simulink subsystem "VehicleElectroThermal"  (R2023a)
settings: Solver=VariableStepAuto  StartTime=0.0  StopTime=10.0  RelTol=1e-3
undefined symbols (not defined in the file): battery, cabin_T_init, coolant_pipe_D, coolant_valve_D_ratio_max, coolant_valve_D_ratio_min, coolant_valve_displacement, vehicleThermal
libraries: fl_lib x199, nesl_utility x54, SimscapeFluids_lib x15, ee_lib x9, sdl_lib x8, slpidlib x3, simulink x2, EmotorLib x2, BatteryCurrentManagement x1
(part 1 of 6)
settings Model: Creator=jjha  LastModifiedBy=jjha
settings OptimizationCC: ReuseModelBlockBuffer=off

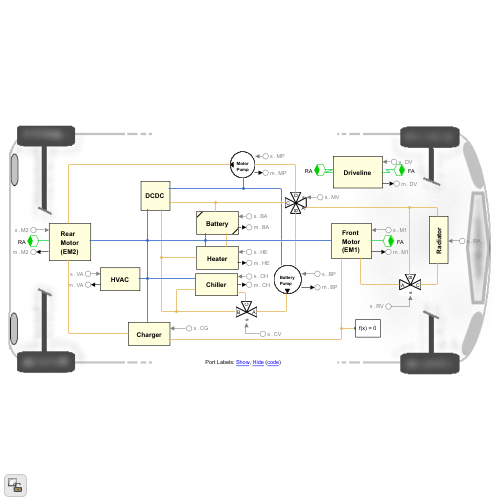
[thumbnail: Simulink's stored preview of the top-level diagram]
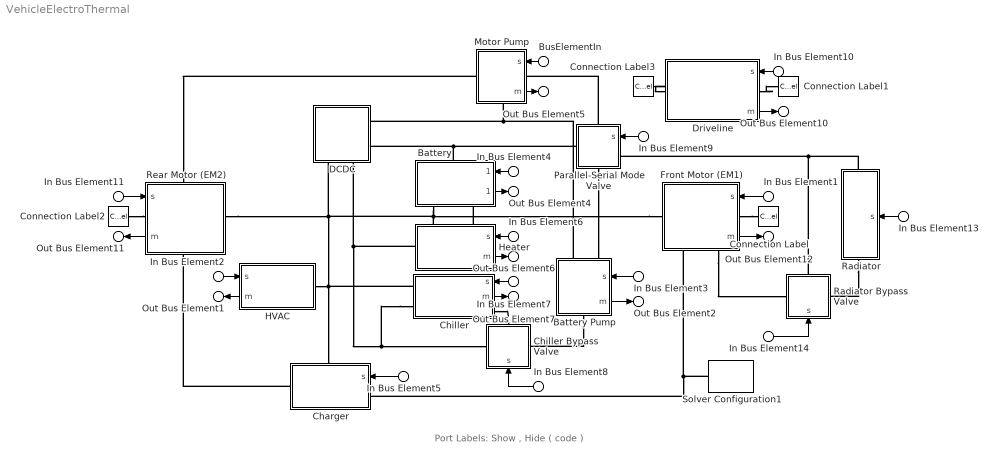
== system VehicleElectroThermal ==
  note: Port Labels: Show , Hide ( code )
  In Bus Element2 : Inport  PortName=s  Element=VA
  In Bus Element3 : Inport  PortName=s  Element=BP
  In Bus Element4 : Inport  PortName=s  Element=BA
  In Bus Element6 : Inport  PortName=s  Element=HE
  In Bus Element7 : Inport  PortName=s  Element=CH
  In Bus Element8 : Inport  PortName=s  Element=CV
  In Bus Element9 : Inport  PortName=s  Element=MV
  In Bus Element10 : Inport  PortName=s  Element=DV
  In Bus Element11 : Inport  PortName=s  Element=M2
  In Bus Element13 : Inport  PortName=s  Element=RA
  In Bus Element14 : Inport  PortName=s  Element=RV
  BusElementIn : Inport  PortName=s  Element=MP
  In Bus Element5 : Inport  PortName=s  Element=CG
  In Bus Element1 : Inport  PortName=s  Element=M1
  Battery : Subsystem  ReferencedSubsystem=BatteryPlantModelLumped_th
      settings: PortSchema="{\"entries\":[{\"content\":{\"sides\":[{\"content\":{\"connectorIds\":[\"In1\",\"Out1\"]},\"type\":\"ConnectorPlacement.EquallySpacedRectSide\",\"uuid\":\"8937d0fc-2bf4-4b6f-a857-82b384a76c94\"},{\"content\":{\"side\":\"RIGHT\"},\"type\":\"ConnectorPlacement.EquallySpacedRectSide\",\"uuid\":\"1ccbeec6-a013-4076-9f98-cb308866a19c\"},{\"content\":{\"connectorIds\":[\"LConn1\"],\"side\":\"TOP\"},\"type\":\"ConnectorPlacement.EquallySpacedRectSide\",\"uuid\":\"77a454e3-c37c-480e-9dd0-9550186f5eb3\"},{\"content\":{\"connectorIds\":[\"RConn1\",\"RConn2\"],\"side\":\"BOTTOM\"},\"type\":\"ConnectorPlacement.EquallySpacedRectSide\",\"uuid\":\"f9a87c6a-7374-41c2-a5df-89d60c915a70\"}]},\"type\":\"ConnectorPlacement.EquallySpacedConnector\",\"uuid\":\"fe008494-fd6d-45a8-bf6b-36872afbad95\"}],\"packageUris\":[\"http://schema.mathworks.com/mf0/Connector/R2020b\"],\"version\":\"1.0\"}"
  Battery Pump : Subsystem  Tag=PublishSubsystem
      settings: PortSchema="{\"entries\":[{\"content\":{\"sides\":[{\"content\":{\"connectorIds\":[\"In1\",\"Out1\"]},\"type\":\"ConnectorPlacement.EquallySpacedRectSide\",\"uuid\":\"f321ff85-78a4-45a4-ab97-f20c5abfaf5e\"},{\"content\":{\"connectorIds\":[],\"side\":\"RIGHT\"},\"type\":\"ConnectorPlacement.EquallySpacedRectSide\",\"uuid\":\"2baf3540-3ef2-4140-8c68-0a1895e3ee25\"},{\"content\":{\"connectorIds\":[\"LConn1\",\"LConn2\"],\"side\":\"TOP\"},\"type\":\"ConnectorPlacement.EquallySpacedRectSide\",\"uuid\":\"1e5b09ba-71c5-41d6-b265-2fb2d783e941\"},{\"content\":{\"connectorIds\":[\"RConn1\"],\"side\":\"BOTTOM\"},\"type\":\"ConnectorPlacement.EquallySpacedRectSide\",\"uuid\":\"998b9f49-32fc-4a08-8ed4-02bb722e6368\"}]},\"type\":\"ConnectorPlacement.EquallySpacedConnector\",\"uuid\":\"4c01441a-ee4a-4858-900a-4caacc6910c3\"}],\"packageUris\":[\"http://schema.mathworks.com/mf0/Connector/R2020b\"],\"version\":\"1.0\"}"
      mask Display:
      | plot(150*cos(linspace(0, 2*pi, 500)), 150*sin(linspace(0, 2*pi, 500)))
      | patch([0 24 -24 0],-1*([100 55 55 100]-1+50),  [0 0 0])
      | %disp(get_param(gcb, 'Name'))
      | disp(['{\bf\fontsize{8}' get_param(gcb, 'Name') '}'], 'texmode','on');
  Charger : Subsystem
      settings: PortSchema="{\"entries\":[{\"content\":{\"sides\":[{\"content\":{\"connectorIds\":[\"In1\",\"LConn1\"]},\"type\":\"ConnectorPlacement.EquallySpacedRectSide\",\"uuid\":\"cb45011f-5d5d-4b7e-92e7-7d115d1e4fd6\"},{\"content\":{\"connectorIds\":[\"RConn1\"],\"side\":\"RIGHT\"},\"type\":\"ConnectorPlacement.EquallySpacedRectSide\",\"uuid\":\"cd67087d-6bbf-411e-9f50-cc3c1f5fce85\"},{\"content\":{\"connectorIds\":[\"LConn2\"],\"side\":\"TOP\"},\"type\":\"ConnectorPlacement.EquallySpacedRectSide\",\"uuid\":\"32ff64c9-862a-431f-9f24-2baf455cdab5\"}]},\"type\":\"ConnectorPlacement.EquallySpacedConnector\",\"uuid\":\"13ffd7d0-36a1-4766-a9dc-2d010b2a8713\"}],\"packageUris\":[\"http://schema.mathworks.com/mf0/Connector/R2020b\"],\"version\":\"1.0\"}"
      mask Display:
      | %disp(get_param(gcb, 'Name'))
      | disp(['{\bf\fontsize{12}' get_param(gcb, 'Name') '}'], 'texmode','on');
  Chiller : Subsystem
      settings: PortSchema="{\"entries\":[{\"content\":{\"sides\":[{\"content\":{\"connectorIds\":[\"LConn1\",\"LConn2\"]},\"type\":\"ConnectorPlacement.EquallySpacedRectSide\",\"uuid\":\"5c01cf01-1aa7-4ead-a658-6b31c847d37c\"},{\"content\":{\"connectorIds\":[\"In1\",\"Out1\",\"RConn1\"],\"side\":\"RIGHT\"},\"type\":\"ConnectorPlacement.EquallySpacedRectSide\",\"uuid\":\"fa598d46-0793-4efa-a9e2-c958f5dfdee6\"},{\"content\":{\"connectorIds\":[],\"side\":\"TOP\"},\"type\":\"ConnectorPlacement.EquallySpacedRectSide\",\"uuid\":\"e82d971a-2580-41ee-87fa-0ab5603b5665\"},{\"content\":{\"connectorIds\":[],\"side\":\"BOTTOM\"},\"type\":\"ConnectorPlacement.EquallySpacedRectSide\",\"uuid\":\"431a910f-738f-40ab-a4d4-f974d0793b92\"}]},\"type\":\"ConnectorPlacement.EquallySpacedConnector\",\"uuid\":\"9f63eeb1-1768-47e0-a5e5-2e43c100d3fd\"}],\"packageUris\":[\"http://schema.mathworks.com/mf0/Connector/R2020b\"],\"version\":\"1.0\"}"
      mask Display:
      | %disp(get_param(gcb, 'Name'))
      | disp(['{\bf\fontsize{12}' get_param(gcb, 'Name') '}'], 'texmode','on');
  Chiller Bypass Valve : Subsystem  Tag=PublishSubsystem
      settings: PortSchema="{\"entries\":[{\"content\":{\"sides\":[{\"content\":{\"connectorIds\":[\"LConn1\"]},\"type\":\"ConnectorPlacement.EquallySpacedRectSide\",\"uuid\":\"3cf8f321-e6af-4e16-922c-cceb23b0b295\"},{\"content\":{\"connectorIds\":[\"In1\"],\"side\":\"RIGHT\"},\"type\":\"ConnectorPlacement.EquallySpacedRectSide\",\"uuid\":\"d134eacd-e7eb-4b63-940a-90eaf4978625\"},{\"content\":{\"connectorIds\":[\"LConn2\"],\"side\":\"TOP\"},\"type\":\"ConnectorPlacement.EquallySpacedRectSide\",\"uuid\":\"57a3d5f7-3b46-4166-b258-196ae00f6810\"},{\"content\":{\"connectorIds\":[\"RConn1\"],\"side\":\"BOTTOM\"},\"type\":\"ConnectorPlacement.EquallySpacedRectSide\",\"uuid\":\"637149da-33c2-49a6-af44-c757a7002402\"}]},\"type\":\"ConnectorPlacement.EquallySpacedConnector\",\"uuid\":\"8ee22012-655b-4352-9f09-996f74687633\"}],\"packageUris\":[\"http://schema.mathworks.com/mf0/Connector/R2020b\"],\"version\":\"1.0\"}"
      mask Display:
      | color('white')
      | plot(100, 100)
      | plot(-100, -100)
      | color('black')
      | 
      | plot([0 -100 -100 0], [0 50 -50 0])
      | plot([0 50 -50 0], [0 100 100 0])
      | plot([0 50 -50 0], [0 -100 -100 0])
  Connection Label : ConnectionLabel  Label=FA
  Connection Label1 : ConnectionLabel  Label=FA
  Connection Label2 : ConnectionLabel  Label=RA
  Connection Label3 : ConnectionLabel  Label=RA
  DCDC : Subsystem
      settings: PortSchema="{\"entries\":[{\"content\":{\"sides\":[{\"content\":{},\"type\":\"ConnectorPlacement.EquallySpacedRectSide\",\"uuid\":\"88f70306-1074-4a2f-bf6e-5266a6fad5cc\"},{\"content\":{\"connectorIds\":[\"RConn1\",\"RConn2\"],\"side\":\"RIGHT\"},\"type\":\"ConnectorPlacement.EquallySpacedRectSide\",\"uuid\":\"c9954f31-88d1-45ba-bccc-746174ca97ad\"},{\"content\":{\"side\":\"TOP\"},\"type\":\"ConnectorPlacement.EquallySpacedRectSide\",\"uuid\":\"3d242faa-6d27-4f03-9691-d9501eee9202\"},{\"content\":{\"connectorIds\":[\"RConn3\",\"RConn4\"],\"side\":\"BOTTOM\"},\"type\":\"ConnectorPlacement.EquallySpacedRectSide\",\"uuid\":\"dbc5cd88-c0c4-43cc-b68d-d7b9b93e8ccf\"}]},\"type\":\"ConnectorPlacement.EquallySpacedConnector\",\"uuid\":\"8b73b678-f81c-41f4-a7f6-152147edfd1f\"}],\"packageUris\":[\"http://schema.mathworks.com/mf0/Connector/R2020b\"],\"version\":\"1.0\"}"
      mask Display:
      | %disp(get_param(gcb, 'Name'))
      | disp(['{\bf\fontsize{12}' get_param(gcb, 'Name') '}'], 'texmode','on');
  Driveline : Subsystem
      settings: PortSchema="{\"entries\":[{\"content\":{\"sides\":[{\"content\":{\"connectorIds\":[\"In1\",\"LConn1\",\"Out1\"]},\"type\":\"ConnectorPlacement.EquallySpacedRectSide\",\"uuid\":\"f321ff85-78a4-45a4-ab97-f20c5abfaf5e\"},{\"content\":{\"connectorIds\":[\"RConn1\"],\"side\":\"RIGHT\"},\"type\":\"ConnectorPlacement.EquallySpacedRectSide\",\"uuid\":\"2baf3540-3ef2-4140-8c68-0a1895e3ee25\"},{\"content\":{\"connectorIds\":[],\"side\":\"TOP\"},\"type\":\"ConnectorPlacement.EquallySpacedRectSide\",\"uuid\":\"1e5b09ba-71c5-41d6-b265-2fb2d783e941\"}]},\"type\":\"ConnectorPlacement.EquallySpacedConnector\",\"uuid\":\"4c01441a-ee4a-4858-900a-4caacc6910c3\"}],\"packageUris\":[\"http://schema.mathworks.com/mf0/Connector/R2020b\"],\"version\":\"1.0\"}"
      mask Display:
      | %disp(get_param(gcb, 'Name'))
      | disp(['{\bf\fontsize{12}' get_param(gcb, 'Name') '}'], 'texmode','on');
  Front Motor (EM1) : Subsystem
      settings: PortSchema="{\"entries\":[{\"content\":{\"sides\":[{\"content\":{\"connectorIds\":[\"In1\",\"LConn1\",\"Out1\"]},\"type\":\"ConnectorPlacement.EquallySpacedRectSide\",\"uuid\":\"7243fc6e-711d-4968-986e-a6ac860e50c1\"},{\"content\":{\"connectorIds\":[\"RConn1\"],\"side\":\"RIGHT\"},\"type\":\"ConnectorPlacement.EquallySpacedRectSide\",\"uuid\":\"18479f7a-8f27-458a-ae71-b38762574ae4\"},{\"content\":{\"connectorIds\":[],\"side\":\"TOP\"},\"type\":\"ConnectorPlacement.EquallySpacedRectSide\",\"uuid\":\"aa936f76-6865-41c5-8414-293bd7d656ce\"},{\"content\":{\"connectorIds\":[\"RConn2\",\"RConn3\"],\"side\":\"BOTTOM\"},\"type\":\"ConnectorPlacement.EquallySpacedRectSide\",\"uuid\":\"336e35a4-9a9a-4631-a8f5-a4d8b8cf9e70\"}]},\"type\":\"ConnectorPlacement.EquallySpacedConnector\",\"uuid\":\"faab3502-7b69-46ce-a6d2-3155f4c3b486\"}],\"packageUris\":[\"http://schema.mathworks.com/mf0/Connector/R2020b\"],\"version\":\"1.0\"}"
      mask Display:
      | %disp(get_param(gcb, 'Name'))
      | disp(['{\bf\fontsize{12}' get_param(gcb, 'Name') '}'], 'texmode','on');
  HVAC : Subsystem
      settings: PortSchema="{\"entries\":[{\"content\":{\"sides\":[{\"content\":{\"connectorIds\":[\"LConn1\"]},\"type\":\"ConnectorPlacement.EquallySpacedRectSide\",\"uuid\":\"f3199610-b7b9-4772-9d43-f46decbe6ee9\"},{\"content\":{\"connectorIds\":[\"In1\",\"Out1\"],\"side\":\"RIGHT\"},\"type\":\"ConnectorPlacement.EquallySpacedRectSide\",\"uuid\":\"92399d3a-435b-4545-8fb9-2408b0c62154\"},{\"content\":{\"connectorIds\":[],\"side\":\"TOP\"},\"type\":\"ConnectorPlacement.EquallySpacedRectSide\",\"uuid\":\"9d5257be-bcde-46da-a005-cbe35149e50d\"},{\"content\":{\"connectorIds\":[],\"side\":\"BOTTOM\"},\"type\":\"ConnectorPlacement.EquallySpacedRectSide\",\"uuid\":\"da7f19de-1e57-4fc2-b5c3-4c1d680ac086\"}]},\"type\":\"ConnectorPlacement.EquallySpacedConnector\",\"uuid\":\"aa27bbb1-a774-4836-83ea-faf9e12779cd\"}],\"packageUris\":[\"http://schema.mathworks.com/mf0/Connector/R2020b\"],\"version\":\"1.0\"}"
      mask Display:
      | %disp(get_param(gcb, 'Name'))
      | disp(['{\bf\fontsize{12}' get_param(gcb, 'Name') '}'], 'texmode','on');
  Heater : Subsystem
      settings: PortSchema="{\"entries\":[{\"content\":{\"sides\":[{\"content\":{\"connectorIds\":[]},\"type\":\"ConnectorPlacement.EquallySpacedRectSide\",\"uuid\":\"f321ff85-78a4-45a4-ab97-f20c5abfaf5e\"},{\"content\":{\"connectorIds\":[\"RConn1\",\"RConn2\"],\"side\":\"RIGHT\"},\"type\":\"ConnectorPlacement.EquallySpacedRectSide\",\"uuid\":\"2baf3540-3ef2-4140-8c68-0a1895e3ee25\"},{\"content\":{\"connectorIds\":[\"Out1\",\"In1\"],\"side\":\"TOP\"},\"type\":\"ConnectorPlacement.EquallySpacedRectSide\",\"uuid\":\"1e5b09ba-71c5-41d6-b265-2fb2d783e941\"},{\"content\":{\"connectorIds\":[\"RConn3\"],\"side\":\"BOTTOM\"},\"type\":\"ConnectorPlacement.EquallySpacedRectSide\",\"uuid\":\"2993c442-350f-4391-ac34-e98798b669d5\"}]},\"type\":\"ConnectorPlacement.EquallySpacedConnector\",\"uuid\":\"4c01441a-ee4a-4858-900a-4caacc6910c3\"}],\"packageUris\":[\"http://schema.mathworks.com/mf0/Connector/R2020b\"],\"version\":\"1.0\"}"
      mask Display:
      | %disp(get_param(gcb, 'Name'))
      | disp(['{\bf\fontsize{12}' get_param(gcb, 'Name') '}'], 'texmode','on');
  Motor Pump : Subsystem  Tag=PublishSubsystem
      settings: PortSchema="{\"entries\":[{\"content\":{\"sides\":[{\"content\":{\"connectorIds\":[\"In1\",\"LConn1\",\"Out1\"]},\"type\":\"ConnectorPlacement.EquallySpacedRectSide\",\"uuid\":\"dafa5c41-979f-4f2b-beb0-03378b6030c3\"},{\"content\":{\"connectorIds\":[\"RConn1\"],\"side\":\"RIGHT\"},\"type\":\"ConnectorPlacement.EquallySpacedRectSide\",\"uuid\":\"2ea2b4cc-bcb0-4b93-915b-9928efecd2a3\"},{\"content\":{\"connectorIds\":[],\"side\":\"TOP\"},\"type\":\"ConnectorPlacement.EquallySpacedRectSide\",\"uuid\":\"e510a9c0-a763-4750-a71a-9698d7ffd631\"},{\"content\":{\"connectorIds\":[\"RConn2\"],\"side\":\"BOTTOM\"},\"type\":\"ConnectorPlacement.EquallySpacedRectSide\",\"uuid\":\"6a9cd967-74c4-4a03-9c08-7c7b4b09ecc0\"}]},\"type\":\"ConnectorPlacement.EquallySpacedConnector\",\"uuid\":\"4a878def-b7f5-448f-823c-c871001bb196\"}],\"packageUris\":[\"http://schema.mathworks.com/mf0/Connector/R2020b\"],\"version\":\"1.0\"}"
      mask Display:
      | plot(150*cos(linspace(0, 2*pi, 500)), 150*sin(linspace(0, 2*pi, 500)))
      | patch([-100 -55 -55 -100]-50, [0 24 -24 0], [0 0 0])
      | %disp(get_param(gcb, 'Name'))
      | disp(['{\bf\fontsize{8}' get_param(gcb, 'Name') '}'], 'texmode','on');
  Parallel-Serial Mode Valve : Subsystem  Tag=PublishSubsystem
      settings: PortSchema="{\"entries\":[{\"content\":{\"sides\":[{\"content\":{\"connectorIds\":[\"LConn1\"]},\"type\":\"ConnectorPlacement.EquallySpacedRectSide\",\"uuid\":\"37aeff26-8a07-411b-9eeb-30a57d0de01e\"},{\"content\":{\"connectorIds\":[\"RConn1\"],\"side\":\"RIGHT\"},\"type\":\"ConnectorPlacement.EquallySpacedRectSide\",\"uuid\":\"5bec464c-49bf-4ce7-bef9-f1dcc380cec5\"},{\"content\":{\"connectorIds\":[\"LConn2\",\"In1\"],\"side\":\"TOP\"},\"type\":\"ConnectorPlacement.EquallySpacedRectSide\",\"uuid\":\"af2a9b5d-b1fd-40d4-a7a1-24f37b8a323f\"},{\"content\":{\"connectorIds\":[\"RConn2\"],\"side\":\"BOTTOM\"},\"type\":\"ConnectorPlacement.EquallySpacedRectSide\",\"uuid\":\"7361a3ef-1473-4ec0-bd8f-80e79015a6c8\"}]},\"type\":\"ConnectorPlacement.EquallySpacedConnector\",\"uuid\":\"019cf393-57f8-4763-b38e-2892ad46a0e9\"}],\"packageUris\":[\"http://schema.mathworks.com/mf0/Connector/R2020b\"],\"version\":\"1.0\"}"
      mask Display:
      | color('white')
      | plot(100, 100)
      | plot(-100, -100)
      | color('black')
      | 
      | plot([0 -100 -100 0], [0 50 -50 0])
      | plot([0 100 100 0], [0 50 -50 0])
      | plot([0 50 -50 0], [0 100 100 0])
      | plot([0 50 -50 0], [0 -100 -100 0])
  Radiator : Subsystem  Tag=PublishSubsystem
      settings: PortSchema="{\"entries\":[{\"content\":{\"sides\":[{\"content\":{\"connectorIds\":[\"LConn1\"]},\"type\":\"ConnectorPlacement.EquallySpacedRectSide\",\"uuid\":\"f321ff85-78a4-45a4-ab97-f20c5abfaf5e\"},{\"content\":{\"connectorIds\":[\"RConn1\"],\"side\":\"RIGHT\"},\"type\":\"ConnectorPlacement.EquallySpacedRectSide\",\"uuid\":\"2baf3540-3ef2-4140-8c68-0a1895e3ee25\"},{\"content\":{\"connectorIds\":[],\"side\":\"TOP\"},\"type\":\"ConnectorPlacement.EquallySpacedRectSide\",\"uuid\":\"1e5b09ba-71c5-41d6-b265-2fb2d783e941\"},{\"content\":{\"connectorIds\":[\"In1\"],\"side\":\"BOTTOM\"},\"type\":\"ConnectorPlacement.EquallySpacedRectSide\",\"uuid\":\"c5239a7c-78e5-4ad8-9ce6-8204a250a1f6\"}]},\"type\":\"ConnectorPlacement.EquallySpacedConnector\",\"uuid\":\"4c01441a-ee4a-4858-900a-4caacc6910c3\"}],\"packageUris\":[\"http://schema.mathworks.com/mf0/Connector/R2020b\"],\"version\":\"1.0\"}"
      mask Display:
      | %disp(get_param(gcb, 'Name'))
      | disp(['{\bf\fontsize{12}' get_param(gcb, 'Name') '}'], 'texmode','on');
  Radiator Bypass Valve : Subsystem  Tag=PublishSubsystem
      settings: PortSchema="{\"entries\":[{\"content\":{\"sides\":[{\"content\":{\"connectorIds\":[\"LConn1\"]},\"type\":\"ConnectorPlacement.EquallySpacedRectSide\",\"uuid\":\"3cf8f321-e6af-4e16-922c-cceb23b0b295\"},{\"content\":{\"connectorIds\":[\"In1\"],\"side\":\"RIGHT\"},\"type\":\"ConnectorPlacement.EquallySpacedRectSide\",\"uuid\":\"d134eacd-e7eb-4b63-940a-90eaf4978625\"},{\"content\":{\"connectorIds\":[\"LConn2\"],\"side\":\"TOP\"},\"type\":\"ConnectorPlacement.EquallySpacedRectSide\",\"uuid\":\"57a3d5f7-3b46-4166-b258-196ae00f6810\"},{\"content\":{\"connectorIds\":[\"RConn1\"],\"side\":\"BOTTOM\"},\"type\":\"ConnectorPlacement.EquallySpacedRectSide\",\"uuid\":\"f8aa24a3-5169-478a-b161-4d226dc0f508\"}]},\"type\":\"ConnectorPlacement.EquallySpacedConnector\",\"uuid\":\"8ee22012-655b-4352-9f09-996f74687633\"}],\"packageUris\":[\"http://schema.mathworks.com/mf0/Connector/R2020b\"],\"version\":\"1.0\"}"
      mask Display:
      | color('white')
      | plot(100, 100)
      | plot(-100, -100)
      | color('black')
      | 
      | plot([0 -100 -100 0], [0 50 -50 0])
      | plot([0 50 -50 0], [0 100 100 0])
      | plot([0 50 -50 0], [0 -100 -100 0])
  Rear Motor (EM2) : Subsystem
      settings: PortSchema="{\"entries\":[{\"content\":{\"sides\":[{\"content\":{\"connectorIds\":[\"LConn1\"]},\"type\":\"ConnectorPlacement.EquallySpacedRectSide\",\"uuid\":\"50b93907-dab5-4c80-8f3d-b9696f7ba561\"},{\"content\":{\"connectorIds\":[\"In1\",\"RConn1\",\"Out1\"],\"side\":\"RIGHT\"},\"type\":\"ConnectorPlacement.EquallySpacedRectSide\",\"uuid\":\"ca5b0fd2-80b7-4a93-a409-39e052d42ed0\"},{\"content\":{\"connectorIds\":[\"LConn2\"],\"side\":\"TOP\"},\"type\":\"ConnectorPlacement.EquallySpacedRectSide\",\"uuid\":\"a20c906c-aee3-4b84-9c3f-344dbfe549ed\"},{\"content\":{\"connectorIds\":[\"RConn2\"],\"side\":\"BOTTOM\"},\"type\":\"ConnectorPlacement.EquallySpacedRectSide\",\"uuid\":\"c8c8c4b4-9dd9-46bd-a7c0-676d6e20cefe\"}]},\"type\":\"ConnectorPlacement.EquallySpacedConnector\",\"uuid\":\"5e07fad4-8c29-4119-b1ea-c96ebc59433e\"}],\"packageUris\":[\"http://schema.mathworks.com/mf0/Connector/R2020b\"],\"version\":\"1.0\"}"
      mask Display:
      | %disp(get_param(gcb, 'Name'))
      | disp(['{\bf\fontsize{12}' get_param(gcb, 'Name') '}'], 'texmode','on');
  Solver Configuration1 : nesl_utility/Solver Configuration  PhysicalDomain=network_engine_domain  SubClassName=solver  LeftPortType=input  RightPortType=generic  Tones=[]  Harmonics=[]  SimulateNoise=off  Profile=off  UseLocalSampling=off  EnableSwitchedLinearOptims=on  FrequencyDomain=off  UseCCode=off  RelTol=0.001  AbsTol=0.001  MinStep=1e-09  ToWorkspace=off  RevertToSquareIcSolve=off  NumHomotopyIterations=100  PhasorMode=off  PhasorModeNumHarmonics=1  ConsistencySolver=NEWTON_XTOL_AFTER_FTOL  IndexReductionMethod=DerivativeReplacement  DoDC=off  ResidualTolerance=1e-09  ConsistencyTolSource=GLOBAL  ConsistencyAbsTol=0.001  ConsistencyRelTol=0.001  ConsistencyTolFactor=0.001  UseLocalSolver=off  LocalSolverChoice=NE_BACKWARD_EULER_ADVANCER  ResolveIndetEquations=on  FunctionEvalNumThread=1  LocalSolverSampleTime=0.001  DoFixedCost=off  MaxNonlinIter=3  MaxModeIter=2  ComputeImpulses=off  ImpulseIterations=2  LinearAlgebra=auto  LinearAlgebraNumThread=0  EquationFormulation=NE_TIME_EF  DelaysMemoryBudget=1024  AutomaticFiltering=on  FilteringTimeConstant=0.001  PartitionStorageMethod=AS_NEEDED  PartitionMemoryBudget=1024  PartitionMethod=ROBUST
  Out Bus Element1 : Outport  PortName=m  Element=VA
  Out Bus Element2 : Outport  PortName=m  Element=BP
  Out Bus Element4 : Outport  PortName=m  Element=BA
  Out Bus Element6 : Outport  PortName=m  Element=HE
  Out Bus Element7 : Outport  PortName=m  Element=CH
  Out Bus Element10 : Outport  PortName=m  Element=DV
  Out Bus Element11 : Outport  PortName=m  Element=M2
  Out Bus Element12 : Outport  PortName=m  Element=M1
  Out Bus Element5 : Outport  PortName=m  Element=MP
  wires:
  In Bus Element2/1 -> HVAC/1(s)
  In Bus Element6/1 -> Heater/1(s)
  In Bus Element4/1 -> Battery/1
  Chiller/1(m) -> Out Bus Element7/1
  In Bus Element7/1 -> Chiller/1(s)
  Battery Pump/1("  m ") -> Out Bus Element2/1
  BusElementIn/1 -> Motor Pump/1(s)
  In Bus Element3/1 -> Battery Pump/1(s)
  Battery/1 -> Out Bus Element4/1
  HVAC/1(m) -> Out Bus Element1/1
  In Bus Element8/1 -> Chiller Bypass Valve/1(s)
  In Bus Element9/1 -> Parallel-Serial Mode Valve/1(s)
  Driveline/1(m) -> Out Bus Element10/1
  In Bus Element10/1 -> Driveline/1(s)
  In Bus Element11/1 -> Rear Motor (EM2)/1(s)
  Rear Motor (EM2)/1(m) -> Out Bus Element11/1
  Front Motor (EM1)/1(m) -> Out Bus Element12/1
  In Bus Element13/1 -> Radiator/1(s)
  In Bus Element14/1 -> Radiator Bypass Valve/1(s)
  In Bus Element5/1 -> Charger/1(s)
  Heater/1(m) -> Out Bus Element6/1
  Motor Pump/1("  m ") -> Out Bus Element5/1
  In Bus Element1/1 -> Front Motor (EM1)/1(s)
  connections:
  Parallel-Serial Mode Valve/LConn2 -- Radiator/RConn1 -- Radiator Bypass Valve/LConn1
  Charger/LConn1 -- Front Motor (EM1)/RConn3 -- Solver Configuration1/RConn1
  Chiller/LConn2 -- Heater/RConn3 -- DCDC/RConn4 -- Chiller Bypass Valve/RConn1
  Parallel-Serial Mode Valve/RConn2 -- DCDC/RConn2 -- Battery/LConn1
  Front Motor (EM1)/RConn1 -- Charger/LConn2 -- HVAC/LConn1 -- Chiller/LConn1 -- Rear Motor (EM2)/LConn1 -- DCDC/RConn3 -- Battery/RConn2 -- Heater/RConn2
  Battery Pump/LConn2 -- Motor Pump/RConn2 -- DCDC/RConn1
  Battery Pump/RConn1 -- Chiller Bypass Valve/LConn2
  Parallel-Serial Mode Valve/RConn1 -- Motor Pump/LConn1
  Motor Pump/RConn1 -- Rear Motor (EM2)/LConn2
  Parallel-Serial Mode Valve/LConn1 -- Battery Pump/LConn1
  Charger/RConn1 -- Rear Motor (EM2)/RConn2
  Connection Label2/LConn1 -- Rear Motor (EM2)/RConn1
  Front Motor (EM1)/LConn1 -- Connection Label/LConn1
  Chiller/RConn1 -- Chiller Bypass Valve/LConn1
  Radiator/LConn1 -- Radiator Bypass Valve/RConn1
  Front Motor (EM1)/RConn2 -- Radiator Bypass Valve/LConn2
  Driveline/LConn1 -- Connection Label1/LConn1
  Connection Label3/LConn1 -- Driveline/RConn1
  Heater/RConn1 -- Battery/RConn1

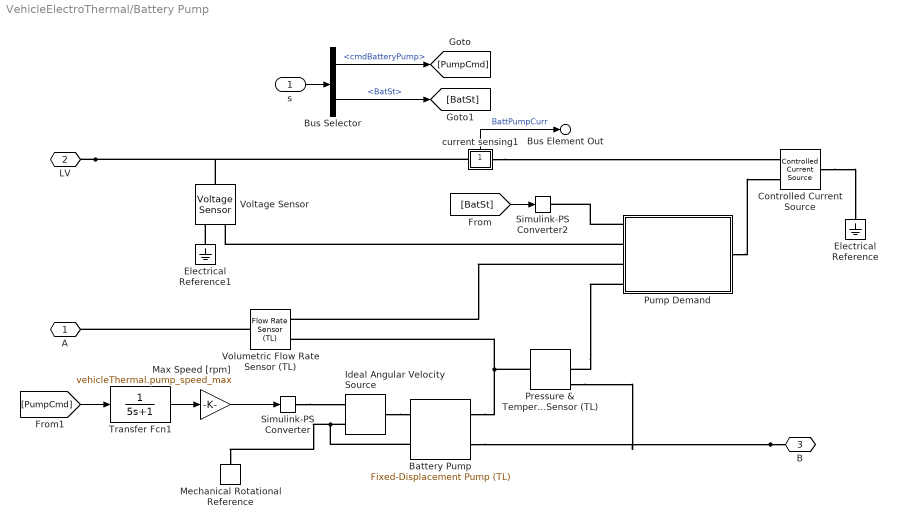
== system VehicleElectroThermal/Battery Pump ==
  s : Inport
  Battery Pump : SimscapeFluids_lib/Thermal Liquid/Pumps & Motors/Fixed-Displacement Pump (TL)  loss_spec=1  displacement=vehicleThermal.pump_displacement l/rev  omega_nominal=0.5 * vehicleThermal.pump_speed_max rpm  p_nominal=0.1 MPa  mu_nominal=0.9 cP  vol_eff_nominal=0.92  mech_eff_nominal=1/(1 + (0.6)/(vehicleThermal.pump_displacement)*0.006283185307179586 + (0.05)/(vehicleThermal.pump_displacement)/(0.1)*0.006283185307179586)  no_load_torque=0.05 N*m  p_diff_eff_TLU=[.1, 1, 2] MPa  omega_eff_TLU=[25, 50, 100, 200, 300, 400] rad/s  vol_eff_TLU=[.816, .908, .954, .977, .981, .984; .325, .663, .831, .916, .925, .946; .137, .568, .78, .892, .893, .91]  mech_eff_TLU=[.996, .996, .996, .996, .996, .996; .988, .989, .989, .989, .989, .99; .981, .981, .982, .982, .983, .984]  p_diff_loss_TLU=[.1, 1, 2] MPa  omega_loss_TLU=[25, 50, 100, 200, 300, 400] rad/s  vol_loss_TLU=[.023, .023, .023, .023, .0285, .032; .0844, .0842, .0845, .084, .1125, .108; .1079, .108, .11, .108, .1605, .18] * 1e-3 m^3/s  mech_loss_TLU=[.002, .002, .002, .002, .002, .002; .0607, .0556, .0556, .0556, .0556, .0505; .1937, .1937, .1833, .1833, .1729, .1626] N*m  vol_eff_min=1e-3  vol_eff_max=1  mech_eff_min=1e-3  mech_eff_max=1  pressure_threshold=1e-3 MPa  omega_threshold=10 rad/s  area=pi * vehicleThermal.coolant_pipe_D^2 / 4 m^2  quadrant_check=0  pump_mode_check=simscape.enum.assert.action.none
  Bus Selector : BusSelector  OutputSignals=cmdBatteryPump,BatSt
  Controlled Current Source : fl_lib/Electrical/Electrical Sources/Controlled Current Source
  Electrical Reference : fl_lib/Electrical/Electrical Elements/Electrical Reference
  Electrical Reference1 : fl_lib/Electrical/Electrical Elements/Electrical Reference
  Ideal Angular Velocity Source : fl_lib/Mechanical/Mechanical Sources/Ideal Angular Velocity Source
  Max Speed [rpm] : Gain  Gain=vehicleThermal.pump_speed_max
  Mechanical Rotational Reference : fl_lib/Mechanical/Rotational Elements/Mechanical Rotational Reference
  Pressure & Temperature Sensor (TL) : fl_lib/Thermal Liquid/Sensors/Pressure & Temperature Sensor (TL)  reference=foundation.enum.MeasurementReference.difference  pressure=true  pressure_spec=foundation.enum.PressureMeasementSpec.Absolute  temperature=true
      settings: InternalSimscapePortConfiguration="{\"Bottom\":[{\"id\":\"T\",\"label\":\"T\",\"type\":\"output\"}],\"Left\":[{\"id\":\"A\",\"label\":\"A\",\"type\":\"foundation.thermal_liquid.thermal_liquid\"}],\"Right\":[{\"id\":\"B\",\"label\":\"B\",\"type\":\"foundation.thermal_liquid.thermal_liquid\"},{\"id\":\"P\",\"label\":\"P\",\"type\":\"output\"}],\"Top\":[]}"
  Pump Demand : Subsystem
  Simulink-PS Converter : nesl_utility/Simulink-PS Converter  PhysicalDomain=network_engine_domain  SubClassName=ps_input  LeftPortType=input  RightPortType=output  PseudoPeriodic=off  Frequencies=[]  NoiseDistribution=none  NoiseParameters=[]  Unit=rpm  AffineConversion=off  FilteringAndDerivatives=provide  SimscapeFilterOrder=1  InputFilterTimeConstant=0.001  UdotUserProvided=0
  Simulink-PS Converter2 : nesl_utility/Simulink-PS Converter  PhysicalDomain=network_engine_domain  SubClassName=ps_input  LeftPortType=input  RightPortType=output  PseudoPeriodic=off  Frequencies=[]  NoiseDistribution=none  NoiseParameters=[]  Unit=1  AffineConversion=off  FilteringAndDerivatives=provide  SimscapeFilterOrder=1  InputFilterTimeConstant=0.001  UdotUserProvided=0
  Transfer Fcn1 : TransferFcn  Denominator=[5 1]
  Voltage Sensor : fl_lib/Electrical/Electrical Sensors/Voltage Sensor
  Volumetric Flow Rate Sensor (TL) : fl_lib/Thermal Liquid/Sensors/Flow Rate Sensor (TL)  mass_flow_measure=false  volumetric_flow_measure=true  energy_flow_measure=false
      settings: InternalSimscapePortConfiguration="{\"Bottom\":[],\"Left\":[{\"id\":\"A\",\"label\":\"A\",\"type\":\"foundation.thermal_liquid.thermal_liquid\"}],\"Right\":[{\"id\":\"B\",\"label\":\"B\",\"type\":\"foundation.thermal_liquid.thermal_liquid\"},{\"id\":\"V\",\"label\":\"V\",\"type\":\"output\"}],\"Top\":[]}"
  current sensing1 : Subsystem
      settings: PortSchema="{\"entries\":[{\"content\":{\"sides\":[{\"content\":{\"connectorIds\":[\"LConn1\"]},\"type\":\"ConnectorPlacement.EquallySpacedRectSide\",\"uuid\":\"be2815b5-7c4b-4452-9f46-9765620d338b\"},{\"content\":{\"connectorIds\":[\"RConn1\"],\"side\":\"RIGHT\"},\"type\":\"ConnectorPlacement.EquallySpacedRectSide\",\"uuid\":\"398ebab2-f4fa-4d00-bf6e-74bf1f6972c5\"},{\"content\":{\"connectorIds\":[\"Out1\"],\"side\":\"TOP\"},\"type\":\"ConnectorPlacement.EquallySpacedRectSide\",\"uuid\":\"f18d5713-17ec-4be9-9072-3e03c5a4f599\"}]},\"type\":\"ConnectorPlacement.EquallySpacedConnector\",\"uuid\":\"966ec05e-6316-4039-8e26-1d6b096cf423\"}],\"packageUris\":[\"http://schema.mathworks.com/mf0/Connector/R2020b\"],\"version\":\"1.0\"}"
  A : PMIOPort  Side=Left
  LV : PMIOPort  Port=2  Side=Left
  B : PMIOPort  Port=3  Side=Right
  Bus Element Out : Outport  PortName=m  Element=BattPumpCurr
  wires:
  Bus Selector/2 -> [BatSt]  "<BatSt>"
  Bus Selector/1 -> [PumpCmd]  "<cmdBatteryPump>"
  [BatSt] -> Simulink-PS Converter2/1
  Transfer Fcn1/1 -> Max Speed [rpm]/1
  Max Speed [rpm]/1 -> Simulink-PS Converter/1
  [PumpCmd] -> Transfer Fcn1/1
  s/1 -> Bus Selector/1
  current sensing1/1("   ") -> Bus Element Out/1  "BattPumpCurr"
  connections:
  Pump Demand/LConn3 -- Volumetric Flow Rate Sensor (TL)/RConn2
  Pump Demand/LConn4 -- Pressure & Temperature Sensor (TL)/RConn2
  Controlled Current Source/LConn1 -- Electrical Reference/LConn1
  Pump Demand/RConn1 -- Controlled Current Source/RConn1
  Pump Demand/LConn1 -- Simulink-PS Converter2/RConn1
  Pump Demand/LConn2 -- Voltage Sensor/RConn1
  Electrical Reference1/LConn1 -- Voltage Sensor/RConn2
  current sensing1/RConn1 -- Controlled Current Source/RConn2
  LV/RConn1 -- Voltage Sensor/LConn1 -- current sensing1/LConn1
  Volumetric Flow Rate Sensor (TL)/LConn1 -- A/RConn1
  Ideal Angular Velocity Source/LConn1 -- Battery Pump/RConn1
  Battery Pump/RConn2 -- Ideal Angular Velocity Source/RConn2 -- Mechanical Rotational Reference/LConn1
  Simulink-PS Converter/RConn1 -- Ideal Angular Velocity Source/RConn1
  B/RConn1 -- Pressure & Temperature Sensor (TL)/RConn1 -- Battery Pump/LConn2
  Pressure & Temperature Sensor (TL)/LConn1 -- Volumetric Flow Rate Sensor (TL)/RConn1 -- Battery Pump/LConn1

== system VehicleElectroThermal/Charger ==
  s : Inport
  Battery CC-CV : BatteryCurrentManagement/Battery CC-CV  MaxCellVoltage=battery.ChargeMaxVolt  Kp=battery.ChargeKp  Ki=battery.ChargerKi  Kaw=battery.ChargerKaw  Kt=1  Ts=-1
      settings: LibrarySourceBlock=batt_sl_lib/Current Management/Battery CC-CV
  Bus Selector4 : BusSelector  OutputSignals=Batt.Relay.RelayChg,Batt.BattSensor.CellVoltMax
  Chargwe Converter mass : fl_lib/Thermal/Thermal Elements/Thermal Mass  mass_type=foundation.enum.constant_variable.constant  mass=1 kg  sp_heat=447 J/kg/K  mass_min=1e-6 kg  num_ports=foundation.enum.numPorts2.one  m_specify=off  m_priority=High  m=1 kg  m_nominal_specify=off  m_nominal_unit=kg  m_nominal_value=1  T_specify=on  T_priority=High  T=vehicleThermal.coolant_T_init K  T_nominal_specify=off  T_nominal_unit=K  T_nominal_value=1  Q_specify=off  Q_priority=None  Q=0 W  Q_nominal_specify=off  Q_nominal_unit=W  Q_nominal_value=1
  Constant Chg Current : Constant  Value=battery.ChargerCC_A
  Controlled Current Source : fl_lib/Electrical/Electrical Sources/Controlled Current Source
  Coolant Jacket : SimscapeFluids_lib/Thermal Liquid/Pipes & Fittings/Pipe (TL)  dynamic_compressibility=1  inertia=0  num_segments=1  pipe_length=0.4 m  cross_section_geometry=fluids.thermal_liquid.pipes_fittings.enum.CrossSectionGeometry.Custom  pipe_diameter=0.1 m  pipe_inner_diameter=0.05 m  pipe_outer_diameter=0.1 m  pipe_width=0.1 m  pipe_height=0.1 m  pipe_major_axis=0.1 m  pipe_minor_axis=0.05 m  pipe_side=0.1 m  pipe_angle=30 deg  area=4 * pi * vehicleThermal.coolant_channel_D^2 / 4 m^2  Dh=vehicleThermal.coolant_channel_D m  wall_spec=1  wall_compliance=1.2e-6 m/MPa  wall_time_constant=0.01 s  elevation_spec=foundation.enum.constant_variable.constant  elevation_gain=0 m  g=9.81 m/s^2  pressure_loss_spec=1  local_pressure_loss_spec=fluids.thermal_liquid.pipes_fittings.enum.LocalLossSpec.AggregateLength  length_add=20 * vehicleThermal.coolant_channel_D * 4 m  loss_coefficient=0.1  roughness_spec=fluids.thermal_liquid.pipes_fittings.enum.RoughnessSpec.Custom  roughness=1.5e-5 m  Re_friction_TLU=[ 400 1000 1.5e+3 3e+3 4e+3 6e+3 1e+4 2e+4 4e+4 6e+4 1e+5 1e+8 ]  friction_factor_TLU=[ 0.264 0.112 0.07099999999999999 0.0417 0.0387 0.0268 0.025 0.0232 0.0226 0.022 0.0214 0.0214 ]  shape_factor=64  Re_lam=100  Re_tur=500  mdot_nominal=[ 0.1 1 ] kg/s  p_diff_nominal=[ 0.001 0.01 ] MPa  mdot_threshold=1e-6 kg/s  heat_transfer_spec=4  mdot_nominal_heat=[ 0.1 1 ] kg/s  T_in_nominal=[ 293.15 293.15 ] K  T_out_nominal=[ 300 300 ] K  p_in_nominal_heat=[ 0.101325 0.101325 ] MPa  T_wall_nominal=[ 303.15 303.15 ] K  a_coeff=0.3  b_Re_power=0.8  c_Pr_power=0.33  Nu_lam=3.66  Re_Colburn_TLU=[ 100 150 1000 ]  Colburn_factor_TLU=[ 0.019 0.013 0.002 ]  Re_Nu_TLU=[ 100 150 1000 ]  Pr_Nu_TLU=[ 1 10 ]  Nu_TLU=[ 3.72 4.21; 3.75 4.44; 4.21 7.15 ]  p0_vec=vehicleThermal.coolant_p_init MPa  T0_vec=vehicleThermal.coolant_T_init K  mdot0=0.1 kg/s
  Electrical Reference : fl_lib/Electrical/Electrical Elements/Electrical Reference
  Ground : Ground
  Heat Flow Source : fl_lib/Thermal/Thermal Sources/Controlled Heat Flow Rate Source
  PS Constant : fl_lib/Physical Signals/Sources/PS Constant  constant=0
  Simulink-PS Converter1 : nesl_utility/Simulink-PS Converter  PhysicalDomain=network_engine_domain  SubClassName=ps_input  LeftPortType=input  RightPortType=output  PseudoPeriodic=off  Frequencies=[]  NoiseDistribution=none  NoiseParameters=[]  Unit=A  AffineConversion=off  FilteringAndDerivatives=provide  SimscapeFilterOrder=2  InputFilterTimeConstant=0.01  UdotUserProvided=0
  Thermal Reference : fl_lib/Thermal/Thermal Elements/Thermal Reference
  Transfer Fcn : TransferFcn  Denominator=[1 1]
  B : PMIOPort  Side=Left
  HV : PMIOPort  Port=2  Side=Left
  A : PMIOPort  Port=3  Side=Right
  wires:
  Transfer Fcn/1 -> Simulink-PS Converter1/1
  Constant Chg Current/1 -> Battery CC-CV/3
  Bus Selector4/2 -> Battery CC-CV/2  "<CellVoltMax>"
  Bus Selector4/1 -> Battery CC-CV/1  "<RelayChg>"
  Battery CC-CV/1 -> Transfer Fcn/1
  Ground/1 -> Battery CC-CV/4
  s/1 -> Bus Selector4/1
  connections:
  Thermal Reference/LConn1 -- Heat Flow Source/RConn2
  PS Constant/RConn1 -- Heat Flow Source/RConn1
  Coolant Jacket/LConn2 -- Chargwe Converter mass/LConn1 -- Heat Flow Source/LConn1
  B/RConn1 -- Coolant Jacket/LConn1
  Electrical Reference/LConn1 -- Controlled Current Source/RConn2
  HV/RConn1 -- Controlled Current Source/LConn1
  Controlled Current Source/RConn1 -- Simulink-PS Converter1/RConn1
  A/RConn1 -- Coolant Jacket/RConn1

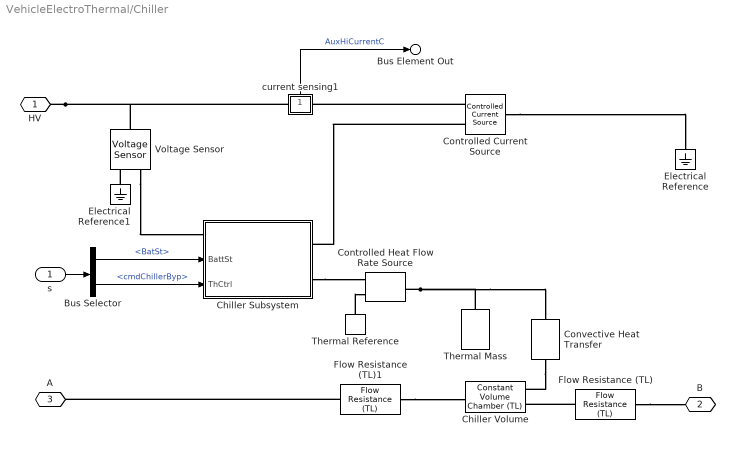
== system VehicleElectroThermal/Chiller ==
  s : Inport
  Bus Selector : BusSelector  OutputSignals=Batt.BatSt,cmdChillerByp
  Chiller Volume : fl_lib/Thermal Liquid/Elements/Constant Volume Chamber (TL)  volume=0.001 m^3  num_ports=foundation.enum.num_ports.two  area_A=pi * vehicleThermal.coolant_pipe_D^2 / 4 m^2  area_B=pi * vehicleThermal.coolant_pipe_D^2 / 4 m^2  area_C=0.01 m^2  area_D=0.01 m^2  p_I_specify=on  p_I_priority=High  p_I=vehicleThermal.coolant_p_init MPa  p_I_nominal_specify=off  p_I_nominal_unit=MPa  p_I_nominal_value=1  T_I_specify=on  T_I_priority=High  T_I=vehicleThermal.coolant_T_init K  T_I_nominal_specify=off  T_I_nominal_unit=K  T_I_nominal_value=1  u_I_specify=off  u_I_priority=None  u_I=83.90600000000001 kJ/kg  u_I_nominal_specify=off  u_I_nominal_unit=kJ/kg  u_I_nominal_value=1  rho_I_specify=off  rho_I_priority=None  rho_I=998.21 kg/m^3  rho_I_nominal_specify=off  rho_I_nominal_unit=kg/m^3  rho_I_nominal_value=1
      settings: InternalSimscapePortConfiguration="{\"Bottom\":[],\"Left\":[{\"id\":\"A\",\"label\":\"A\",\"type\":\"foundation.thermal_liquid.thermal_liquid\"},{\"id\":\"H\",\"label\":\"H\",\"type\":\"foundation.thermal.thermal\"}],\"Right\":[{\"id\":\"B\",\"label\":\"B\",\"type\":\"foundation.thermal_liquid.thermal_liquid\"}],\"Top\":[]}"
  Chiller Subsystem : Subsystem
      settings: PortSchema="{\"entries\":[{\"content\":{\"sides\":[{\"content\":{\"connectorIds\":[\"LConn1\",\"In1\",\"In2\"]},\"type\":\"ConnectorPlacement.EquallySpacedRectSide\",\"uuid\":\"d995acd0-973b-4873-b050-eaa71c2c53f5\"},{\"content\":{\"connectorIds\":[\"RConn1\",\"RConn2\"],\"side\":\"RIGHT\"},\"type\":\"ConnectorPlacement.EquallySpacedRectSide\",\"uuid\":\"f40dc2d9-a9a2-427c-8e3f-65ba63c73559\"},{\"content\":{\"connectorIds\":[],\"side\":\"TOP\"},\"type\":\"ConnectorPlacement.EquallySpacedRectSide\",\"uuid\":\"1868aaf5-b9f5-4fdb-94e9-4b9189d403a5\"}]},\"type\":\"ConnectorPlacement.EquallySpacedConnector\",\"uuid\":\"c13a0ccf-549d-47cf-8e66-a96ce55255c8\"}],\"packageUris\":[\"http://schema.mathworks.com/mf0/Connector/R2020b\"],\"version\":\"1.0\"}"
  Controlled Current Source : fl_lib/Electrical/Electrical Sources/Controlled Current Source
  Controlled Heat Flow Rate Source : fl_lib/Thermal/Thermal Sources/Controlled Heat Flow Rate Source
  Convective Heat Transfer : fl_lib/Thermal/Thermal Elements/Convective Heat Transfer  thermal_type=foundation.enum.constant_variable.constant  area=1 m^2  heat_tr_coeff=200 W/(m^2 * K)  min_heat_tr_coeff=1e-3 W/(K*m^2)  T_specify=off  T_priority=None  T=0 K  T_nominal_specify=off  T_nominal_unit=K  T_nominal_value=1  Q_specify=off  Q_priority=None  Q=0 W  Q_nominal_specify=off  Q_nominal_unit=W  Q_nominal_value=1
  Electrical Reference : fl_lib/Electrical/Electrical Elements/Electrical Reference
  Electrical Reference1 : fl_lib/Electrical/Electrical Elements/Electrical Reference
  Flow Resistance (TL) : fl_lib/Thermal Liquid/Elements/Flow Resistance (TL)  delta_p_nominal=2e-4 MPa  mdot_nominal=0.15 kg/s  area=pi * vehicleThermal.coolant_pipe_D^2 / 4 m^2  laminar_fraction=1e-3
  Flow Resistance (TL)1 : fl_lib/Thermal Liquid/Elements/Flow Resistance (TL)  delta_p_nominal=2e-4 MPa  mdot_nominal=0.15 kg/s  area=pi * vehicleThermal.coolant_pipe_D^2 / 4 m^2  laminar_fraction=1e-3
  Thermal Mass : fl_lib/Thermal/Thermal Elements/Thermal Mass  mass_type=foundation.enum.constant_variable.constant  mass=2 kg  sp_heat=447 J/kg/K  mass_min=1e-6 kg  num_ports=foundation.enum.numPorts2.one  m_specify=off  m_priority=High  m=1 kg  m_nominal_specify=off  m_nominal_unit=kg  m_nominal_value=1  T_specify=on  T_priority=High  T=vehicleThermal.coolant_T_init K  T_nominal_specify=off  T_nominal_unit=K  T_nominal_value=1  Q_specify=off  Q_priority=None  Q=0 W  Q_nominal_specify=off  Q_nominal_unit=W  Q_nominal_value=1
  Thermal Reference : fl_lib/Thermal/Thermal Elements/Thermal Reference
  Voltage Sensor : fl_lib/Electrical/Electrical Sensors/Voltage Sensor
  current sensing1 : Subsystem
      settings: PortSchema="{\"entries\":[{\"content\":{\"sides\":[{\"content\":{\"connectorIds\":[\"LConn1\"]},\"type\":\"ConnectorPlacement.EquallySpacedRectSide\",\"uuid\":\"be2815b5-7c4b-4452-9f46-9765620d338b\"},{\"content\":{\"connectorIds\":[\"RConn1\"],\"side\":\"RIGHT\"},\"type\":\"ConnectorPlacement.EquallySpacedRectSide\",\"uuid\":\"398ebab2-f4fa-4d00-bf6e-74bf1f6972c5\"},{\"content\":{\"connectorIds\":[\"Out1\"],\"side\":\"TOP\"},\"type\":\"ConnectorPlacement.EquallySpacedRectSide\",\"uuid\":\"f18d5713-17ec-4be9-9072-3e03c5a4f599\"}]},\"type\":\"ConnectorPlacement.EquallySpacedConnector\",\"uuid\":\"966ec05e-6316-4039-8e26-1d6b096cf423\"}],\"packageUris\":[\"http://schema.mathworks.com/mf0/Connector/R2020b\"],\"version\":\"1.0\"}"
  HV : PMIOPort  Side=Left
  B : PMIOPort  Port=2  Side=Left
  A : PMIOPort  Port=3  Side=Right
  Bus Element Out : Outport  PortName=m  Element=ChillerCurrent
  wires:
  s/1 -> Bus Selector/1
  current sensing1/1("   ") -> Bus Element Out/1  "AuxHiCurrentC"
  Bus Selector/2 -> Chiller Subsystem/2(ThCtrl)  "<cmdChillerByp>"
  Bus Selector/1 -> Chiller Subsystem/1(BattSt)  "<BatSt>"
  connections:
  Voltage Sensor/RConn1 -- Chiller Subsystem/LConn1
  Electrical Reference1/LConn1 -- Voltage Sensor/RConn2
  Controlled Current Source/RConn1 -- Chiller Subsystem/RConn1
  Thermal Reference/LConn1 -- Controlled Heat Flow Rate Source/RConn2
  Convective Heat Transfer/RConn1 -- Chiller Volume/LConn2
  Flow Resistance (TL)1/RConn1 -- Chiller Volume/RConn1
  Controlled Heat Flow Rate Source/LConn1 -- Convective Heat Transfer/LConn1 -- Thermal Mass/LConn1
  Flow Resistance (TL)/RConn1 -- B/RConn1
  Flow Resistance (TL)/LConn1 -- Chiller Volume/LConn1
  Chiller Subsystem/RConn2 -- Controlled Heat Flow Rate Source/RConn1
  Controlled Current Source/LConn1 -- Electrical Reference/LConn1
  HV/RConn1 -- Voltage Sensor/LConn1 -- current sensing1/LConn1
  Controlled Current Source/RConn2 -- current sensing1/RConn1
  Flow Resistance (TL)1/LConn1 -- A/RConn1

== system VehicleElectroThermal/Chiller Bypass Valve ==
  s : Inport
  Chiller Bypass Valve : SimscapeFluids_lib/Thermal Liquid/Valves & Orifices/Directional Control Valves/3-Way Directional Valve (TL)  open_orifices_pos=fluids.thermal_liquid.valves.directional_control_valves.enum.OpenOrifices3Way.PA  open_orifices_neg=fluids.thermal_liquid.valves.directional_control_valves.enum.OpenOrifices3Way.AT  area_spec=fluids.thermal_liquid.valves.directional_control_valves.enum.area_spec.identical  valve_spec=fluids.thermal_liquid.valves.enum.orifice_spec.linear  del_S_max=vehicleThermal.coolant_valve_displacement-(vehicleThermal.coolant_valve_displacement)*(pi * (vehicleThermal.coolant_valve_D_ratio_min*vehicleThermal.coolant_pipe_D)^2 / 4)/(pi * (vehicleThermal.coolant_valve_D_ratio_max*vehicleThermal.coolant_pipe_D)^2 / 4) m  area_max=pi * (vehicleThermal.coolant_valve_D_ratio_max*vehicleThermal.coolant_pipe_D)^2 / 4 m^2  del_S_TLU=[0 0.002 0.004 0.007 0.017] m  valve_area_TLU=[1e-09, 2.0352e-07, 4.0736e-05, .00011438, .00034356] m^2  del_S_flow_TLU=[0 0.002 0.004 0.007 0.017] m  p_diff_TLU=[-.1, .3, .5, .7] MPa  vol_flow_TLU=1e-3 * [1.7e-05, 2e-05, 2.6e-05; .0035, .0045, .0053; .7, .9, 1.06; 1.96, 2.5, 3; 6, 7.7, 9.13] m^3/s  mdot_TLU=[-1e-05, 1.7e-05, 2e-05, 2.6e-05; -.002, .0035, .0045, .0053; -.4, .7, .9, 1.06; -1.13, 1.96, 2.5, 3; -3.45, 6, 7.7, 9.13] kg/s  T_ref_in=293.15 K  p_ref_in=0.101325 MPa  area_leak=pi * (vehicleThermal.coolant_valve_D_ratio_min*vehicleThermal.coolant_pipe_D)^2 / 4 m^2  Cd=0.7  Re_c=12  smoothing_factor=0.01  pressure_recovery=simscape.enum.onoff.on  area=pi * vehicleThermal.coolant_pipe_D^2 / 4 m^2  S_max_PA=(vehicleThermal.coolant_valve_displacement)*(pi * (vehicleThermal.coolant_valve_D_ratio_min*vehicleThermal.coolant_pipe_D)^2 / 4)/(pi * (vehicleThermal.coolant_valve_D_ratio_max*vehicleThermal.coolant_pipe_D)^2 / 4) - (vehicleThermal.coolant_valve_offset) + vehicleThermal.coolant_valve_displacement-(vehicleThermal.coolant_valve_displacement)*(pi * (vehicleThermal.coolant_valve_D_ratio_min*vehicleThermal.coolant_pipe_D)^2 / 4)/(pi * (vehicleThermal.coolant_valve_D_ratio_max*vehicleThermal.coolant_pipe_D)^2 / 4) m  del_S_max_PA=coolant_valve_displacement-(coolant_valve_displacement)*(pi * (coolant_valve_D_ratio_min*coolant_pipe_D)^2 / 4)/(pi * (coolant_valve_D_ratio_max*coolant_pipe_D)^2 / 4) m  area_max_PA=pi * (coolant_valve_D_ratio_max*coolant_pipe_D)^2 / 4 m^2  del_S_TLU_PA=[0 0.002 0.004 0.007 0.017] m  valve_area_TLU_PA=[1e-09, 2.0352e-07, 4.0736e-05, .00011438, .00034356] m^2  del_S_flow_TLU_PA=[0 0.002 0.004 0.007 0.017] m  p_diff_TLU_PA=[-.1, .3, .5, .7] MPa  vol_flow_TLU_PA=1e-3 * [1.7e-05, 2e-05, 2.6e-05; .0035, .0045, .0053; .7, .9, 1.06; 1.96, 2.5, 3; 6, 7.7, 9.13] m^3/s  mdot_TLU_PA=[-1e-05, 1.7e-05, 2e-05, 2.6e-05; -.002, .0035, .0045, .0053; -.4, .7, .9, 1.06; -1.13, 1.96, 2.5, 3; -3.45, 6, 7.7, 9.13] kg/s  S_max_AT=-(vehicleThermal.coolant_valve_displacement)*(pi * (vehicleThermal.coolant_valve_D_ratio_min*vehicleThermal.coolant_pipe_D)^2 / 4)/(pi * (vehicleThermal.coolant_valve_D_ratio_max*vehicleThermal.coolant_pipe_D)^2 / 4) + (vehicleThermal.coolant_valve_offset) - (vehicleThermal.coolant_valve_displacement-(vehicleThermal.coolant_valve_displacement)*(pi * (vehicleThermal.coolant_valve_D_ratio_min*vehicleThermal.coolant_pipe_D)^2 / 4)/(pi * (vehicleThermal.coolant_valve_D_ratio_max*vehicleThermal.coolant_pipe_D)^2 / 4)) m  del_S_max_AT=coolant_valve_displacement-(coolant_valve_displacement)*(pi * (coolant_valve_D_ratio_min*coolant_pipe_D)^2 / 4)/(pi * (coolant_valve_D_ratio_max*coolant_pipe_D)^2 / 4) m  area_max_AT=pi * (coolant_valve_D_ratio_max*coolant_pipe_D)^2 / 4 m^2  del_S_TLU_AT=[0 0.002 0.004 0.007 0.017] m  valve_area_TLU_AT=[1e-09, 2.0352e-07, 4.0736e-05, .00011438, .00034356] m^2  del_S_flow_TLU_AT=[0 0.002 0.004 0.007 0.017] m  p_diff_TLU_AT=[-.1, .3, .5, .7] MPa  vol_flow_TLU_AT=1e-3 * [1.7e-05, 2e-05, 2.6e-05; .0035, .0045, .0053; .7, .9, 1.06; 1.96, 2.5, 3; 6, 7.7, 9.13] m^3/s  mdot_TLU_AT=[-1e-05, 1.7e-05, 2e-05, 2.6e-05; -.002, .0035, .0045, .0053; -.4, .7, .9, 1.06; -1.13, 1.96, 2.5, 3; -3.45, 6, 7.7, 9.13] kg/s  S_max_PT=2.5e-3 m  del_S_max_PT=0.005 m  area_max_PT=1e-4 m^2  del_S_TLU_PT=[0, .002, .004, .007, .017] m  valve_area_TLU_PT=[1e-09, 2.0352e-07, 4.0736e-05, .00011438, .00034356] m^2  del_S_flow_TLU_PT=[0, .002, .004, .007, .017] m  p_diff_TLU_PT=[.3, .5, .7] MPa  vol_flow_TLU_PT=1e-3 * [1.7e-05, 2e-05, 2.6e-05; .0035, .0045, .0053; .7, .9, 1.06; 1.96, 2.5, 3; 6, 7.7, 9.13] m^3/s  mdot_TLU_PT=[1.7e-05, 2e-05, 2.6e-05; .0035, .0045, .0053; .7, .9, 1.06; 1.96, 2.5, 3; 6, 7.7, 9.13] kg/s
      settings: InternalSimscapePortConfiguration="{\"Bottom\":[],\"Left\":[{\"id\":\"A\",\"label\":\"A\",\"type\":\"foundation.thermal_liquid.thermal_liquid\"}],\"Right\":[{\"id\":\"S\",\"label\":\"S\",\"type\":\"input\"},{\"id\":\"P\",\"label\":\"P\",\"type\":\"foundation.thermal_liquid.thermal_liquid\"},{\"id\":\"T\",\"label\":\"T\",\"type\":\"foundation.thermal_liquid.thermal_liquid\"}],\"Top\":[]}"
  Flow Resistance (TL) : fl_lib/Thermal Liquid/Elements/Flow Resistance (TL)  delta_p_nominal=0.001 MPa  mdot_nominal=0.3 kg/s  area=pi * vehicleThermal.coolant_pipe_D^2 / 4 m^2  laminar_fraction=1e-3
  Valve Control : Subsystem
  C : PMIOPort  Side=Left
  A : PMIOPort  Port=2  Side=Left
  B : PMIOPort  Port=3  Side=Right
  wires:
  s/1 -> Valve Control/1(ThCtrl)
  connections:
  Flow Resistance (TL)/LConn1 -- Chiller Bypass Valve/RConn2
  A/RConn1 -- Chiller Bypass Valve/LConn1
  Valve Control/RConn1 -- Chiller Bypass Valve/RConn1
  C/RConn1 -- Chiller Bypass Valve/RConn3
  Flow Resistance (TL)/RConn1 -- B/RConn1
